simulink model "RLC_Circuit"  (R2022a)
settings: Solver=ode45  StartTime=0.0  StopTime=0.02  RelTol=1e-3
settings Model: Creator=Kieran  LastModifiedBy=Kieran

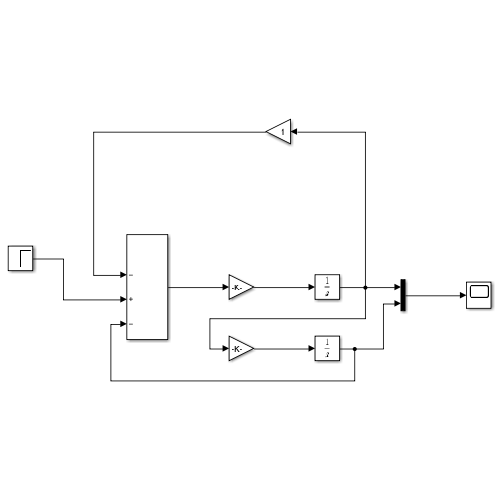
[thumbnail: Simulink's stored preview of the top-level diagram]
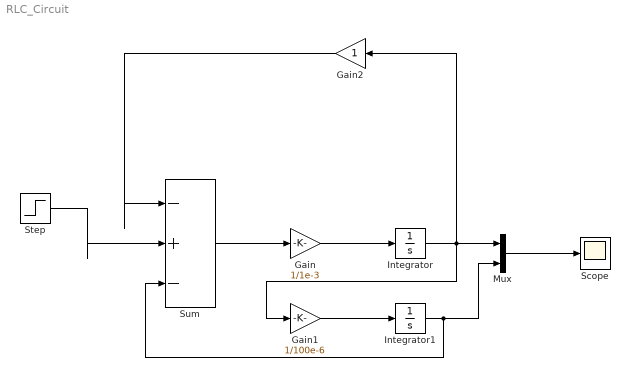
== system RLC_Circuit ==
  Gain : Gain  Gain=1/1e-3
  Gain1 : Gain  Gain=1/100e-6
  Gain2 : Gain
  Integrator : Integrator
  Integrator1 : Integrator
  Mux : Mux  Inputs=2
  Scope : Scope
  Step : Step  Time=0  Before=10  After=10  SampleTime=0
  Sum : Sum  Inputs=|-+-
  wires:
  Step/1 -> Sum/2
  Sum/1 -> Gain/1
  Integrator/1 -> Gain2/1, Gain1/1, Mux/1
  Gain/1 -> Integrator/1
  Mux/1 -> Scope/1
  Gain1/1 -> Integrator1/1
  Gain2/1 -> Sum/1
  Integrator1/1 -> Sum/3, Mux/2
